simulink model "Opt_AW"  (R2016b)
settings: Solver=ode5  StartTime=0.0  StopTime=0.5  FixedStep=1e-5  MaxStep=5e-5  MinStep=1e-14  RelTol=1e-12  AbsTol=1e-12  EnableMultiTasking=on
values from neighbouring files (symbols this model uses):
  Af = [-26.5690192801 -2234.33779773 310.893754564 -36.2178332501 -112.152704923 135.866328159 -2.70290332775 -29.6286077383 -16.8207473121 1.8274424151 1.9808708767 -2.22425140753 ... (324 elements, 18x18)]    [all_vars.mat]    (also in main_matlab.m = sysc_full.A)
  Ak = [-684.448289528 -1838.02275685 -245.449466562 329.096259703 75.0041195994 3.82706915823 1217.45439277 -372.514986285 172.466831781 194.781937877 259.855231872 9.91843311764 ... (36 elements, 6x6)]    [all_vars.mat]    (also in controller.mat; main_matlab.m = rlqg.A)
  Bf = [163.35574211 -241.976546968 7.0786716734 -21.2065400752 28.7342734194 408.148266694 31.9999619754 178.159551463 -43.7162224614 14.7755554248 200.513279483 -78.5518542603 ... (36 elements, 18x2)]    [all_vars.mat]    (also in main_matlab.m = sysc_full.B(:,1:2))
  Bk = [-81.4819421286  292.924842313; 300.719243091  42.9479523448; -1170.07972993  -732.159461163; 254.772556959  876.819017487; -390.775314978  123.207611647; -45.8372700719  -43.6955248003]    [all_vars.mat]    (also in controller.mat; main_matlab.m = rlqg.B)
  Cf = [-0.282177127462 0.00836238608882 0.276772202181 -0.0961493631367 -0.0606298017199 0.152574299346 0.123302117864 -0.0217617685764 -0.0652712719626 0.235533425991 -0.265874482692 -0.1840424473 ... (36 elements, 2x18)]    [all_vars.mat]    (also in main_matlab.m = sysc_full.C)
  Ck = [1.54009703707  -0.116962618999  -2.09402947011  -5.28066592983  -1.24392730196  -9.20557682957; -8.80971369205  -3.43163961296  -5.78337983754  7.01971817871  -0.897914006953  -9.71423447702]    [all_vars.mat]    (also in controller.mat; main_matlab.m = rlqg.C)
  Dk = [0  0; 0  0]    [all_vars.mat]    (also in controller.mat; main_matlab.m = rlqg.D)
  Hf = [4.61714302416 2.86223612891 16.5002041415 6.0488685566 1.65239679346 8.71139933515 -20.0964152161 -20.8789999506 -35.4081292702 -15.995581391 7.45467044913 19.9918454326 ... (18 elements, 18x1)]    [all_vars.mat]    (also in main_matlab.m = sysc_full.B(:,4))
  nu = numel(Bp)/np    [main_matlab.m]    (also in opt_obj.m = 2)
  theta = [-0.971465582713  -0.0327343122718; -0.00881803365077  -0.978705545356; -0.00044221075776  -0.00968397090612; -0.000950054796778  0.00118153214645]    [all_vars.mat]    (also in main_matlab.m = L*inv(U))
libraries: cstblocks x2
settings Model: Creator=p4wp4w  LastModifiedBy=ABLAH
settings DataIOCC: LimitDataPoints=on  SaveFormat=Array
settings OptimizationCC: LifeSpan=inf
settings DebuggingCC: SFUnexpectedBacktrackingDiag=warning  SFNoUnconditionalDefaultTransitionDiag=warning  SFExecutionAtInitializationDiag=none
settings HardwareCC: ProdBitPerPointer=32  ProdBitPerSizeT=32  ProdBitPerPtrDiffT=32  ProdLargestAtomicFloat=None  ProdIntDivRoundTo=Undefined  ProdEndianess=Unspecified  ProdWordSize=32  ProdHWDeviceType=32-bit Generic
settings ModelReferenceCC: PropagateSignalLabelsOutOfModel=off
settings GRTTargetCC: TargetLangStandard=C89/C90 (ANSI)  GeneratePreprocessorConditionals=Disable all
settings ConfigComp: CovMetricSettings=dw  CovHtmlReporting=on  CovSaveCumulativeToWorkspaceVar=on  CovSaveSingleToWorkspaceVar=on  CovExternalEMLEnable=off

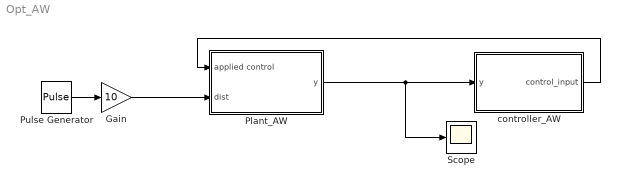
== system Opt_AW ==
  Gain : Gain  Gain=10
  Plant_AW : Subsystem
  Pulse Generator : DiscretePulseGenerator  PulseType=Time based  Period=0.5  PulseWidth=10
  Scope : Scope
  controller_AW : Subsystem
  wires:
  Plant_AW/1(y) -> Scope/1, controller_AW/1(y)
  controller_AW/1("control_input ") -> Plant_AW/1(applied control)
  Pulse Generator/1 -> Gain/1
  Gain/1 -> Plant_AW/2(dist)

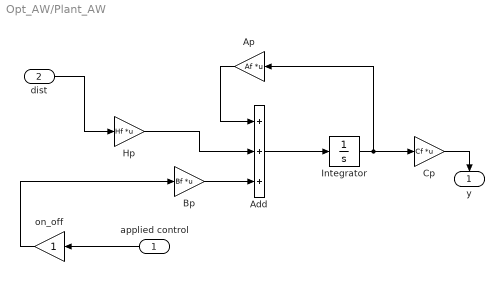
== system Opt_AW/Plant_AW ==
  applied control : Inport
  dist : Inport  Port=2
  Add : Sum  Inputs=+++
  Ap : Gain  Gain=Af  Multiplication=Matrix(K*u)
  Bp : Gain  Gain=Bf  Multiplication=Matrix(K*u)
  Cp : Gain  Gain=Cf  Multiplication=Matrix(K*u)
  Hp : Gain  Gain=Hf  Multiplication=Matrix(K*u)
  Integrator : Integrator
  on_off : Gain
  y : Outport
  wires:
  Add/1 -> Integrator/1
  Cp/1 -> y/1
  Hp/1 -> Add/2
  on_off/1 -> Bp/1
  Integrator/1 -> Cp/1, Ap/1
  Ap/1 -> Add/1
  Bp/1 -> Add/3
  dist/1 -> Hp/1
  applied control/1 -> on_off/1

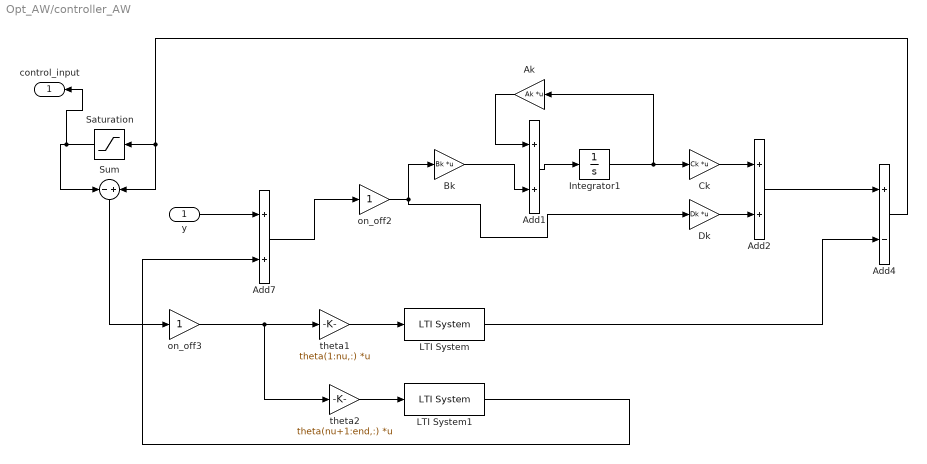
== system Opt_AW/controller_AW ==
  y : Inport
  Add1 : Sum
  Add2 : Sum
  Add4 : Sum  Inputs=+-
  Add7 : Sum
  Ak : Gain  Gain=Ak  Multiplication=Matrix(K*u)
  Bk : Gain  Gain=Bk  Multiplication=Matrix(K*u)
  Ck : Gain  Gain=Ck  Multiplication=Matrix(K*u)
  Dk : Gain  Gain=Dk  Multiplication=Matrix(K*u)
  Integrator1 : Integrator
  LTI System : cstblocks/LTI System  sys=F1  IC=[]
  LTI System1 : cstblocks/LTI System  sys=F2  IC=[]
  Saturation : Saturate  UpperLimit=2  LowerLimit=-2
  Sum : Sum  Inputs=-|+
  on_off2 : Gain
  on_off3 : Gain
  theta1 : Gain  Gain=theta(1:nu,:)  Multiplication=Matrix(K*u)
  theta2 : Gain  Gain=theta(nu+1:end,:)  Multiplication=Matrix(K*u)
  "control_input " : Outport
  wires:
  Ck/1 -> Add2/1
  Add1/1 -> Integrator1/1
  Ak/1 -> Add1/1
  Bk/1 -> Add1/2
  Integrator1/1 -> Ck/1, Ak/1
  Dk/1 -> Add2/2
  on_off2/1 -> Dk/1, Bk/1
  Add2/1 -> Add4/1
  y/1 -> Add7/1
  Add7/1 -> on_off2/1
  LTI System/1 -> Add4/2
  LTI System1/1 -> Add7/2
  theta1/1 -> LTI System/1
  theta2/1 -> LTI System1/1
  on_off3/1 -> theta1/1, theta2/1
  Add4/1 -> Sum/2, Saturation/1
  Saturation/1 -> "control_input "/1, Sum/1
  Sum/1 -> on_off3/1
